simulink model "fuzzy_5"  (R2021a)
settings: Solver=VariableStepAuto  StartTime=0.0  StopTime=10.0  RelTol=1e-3
libraries: fuzblock x1
settings Model: SimulationMode=rapid-accelerator  Creator=USUARIO  LastModifiedBy=USUARIO

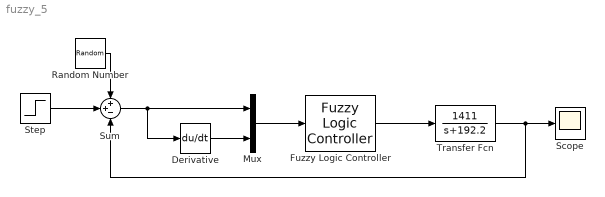
== system fuzzy_5 ==
  Derivative : Derivative
  Fuzzy Logic Controller : fuzblock/Fuzzy Logic  Controller  FIS='fuzzy_5.fis'  OutputSampleNumber=101  DataType=double  FuzzifiedInputs=off  RuleFiringStrengths=off  RuleOutputs=off  AggregatedOutputs=off  SimulateUsing=Interpreted execution  OutOfRangeInputValueMessage=warning  NoRuleFiredMessage=warning  EmptyOutputFuzzySetMessage=warning
  Mux : Mux  Inputs=2
  Random Number : RandomNumber  SampleTime=0.1
  Scope : Scope
  Step : Step  After=100  SampleTime=0
  Sum : Sum  Inputs=++-
  Transfer Fcn : TransferFcn  Numerator=[1411]  Denominator=[1 192.2]
  wires:
  Mux/1 -> Fuzzy Logic Controller/1
  Derivative/1 -> Mux/2
  Transfer Fcn/1 -> Sum/3, Scope/1
  Fuzzy Logic Controller/1 -> Transfer Fcn/1
  Sum/1 -> Derivative/1, Mux/1
  Step/1 -> Sum/2
  Random Number/1 -> Sum/1
